simulink model "MPC_vs_LQR"  (R2014b)
settings: Solver=ode45  StartTime=0.0  StopTime=T_sim  RelTol=1e-3
values from neighbouring files (symbols this model uses):
  N = 100    [cessna.m]
  Q = eye(4)    [cessna.m]
  R = 1    [cessna.m]
  set_point = [0; 0; 0; 0]    [cessna.m]
  sys_discrete = c2d(sys, Ts)    [cessna.m]
  Ts = 0.1    [cessna.m]
  u_max_simulink = inf    [cessna.m]
  u_min_simulink = -inf    [cessna.m]
  x0 = [0; 0; 0; 10]    [cessna.m]
undefined symbols (not defined in the file or in its folder): Kdlqr, MPC_controller, S
settings Model: Creator=lele  LastModifiedBy=lele

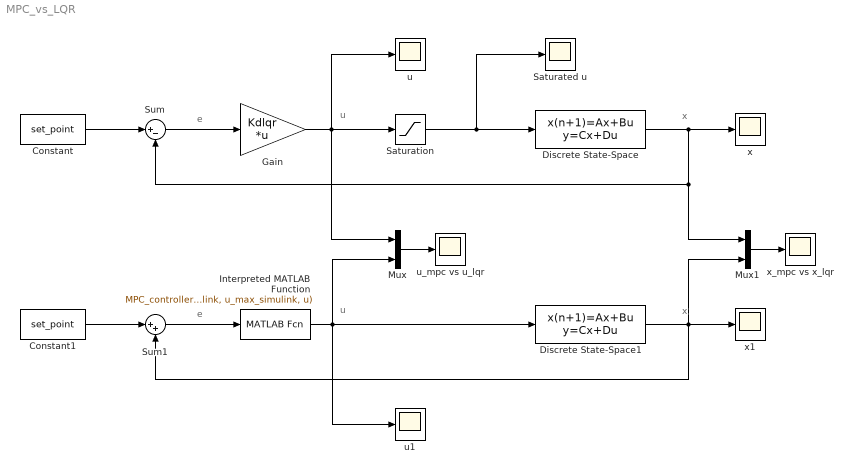
== system MPC_vs_LQR ==
  note: x
  note: u
  note: e
  note: x
  note: u
  note: e
  Constant : Constant  Value=set_point
  Constant1 : Constant  Value=set_point
  Discrete State-Space : DiscreteStateSpace  A=sys_discrete.a  B=sys_discrete.b  C=eye(4)  D=zeros(4, 1)  X0=x0  SampleTime=Ts
  Discrete State-Space1 : DiscreteStateSpace  A=sys_discrete.a  B=sys_discrete.b  C=eye(4)  D=zeros(4, 1)  X0=x0  SampleTime=Ts
  Gain : Gain  Gain=Kdlqr  Multiplication=Matrix(K*u)
  Interpreted MATLAB Function : MATLABFcn  MATLABFcn=MPC_controller(sys_discrete.a, sys_discrete.b, Q, R, S, N, u_min_simulink, u_max_simulink, u)
  Mux : Mux  Inputs=2
  Mux1 : Mux  Inputs=2
  Saturated u : Scope
      settings: SaveName=ScopeData2
  Saturation : Saturate  UpperLimit=u_max_simulink  LowerLimit=u_min_simulink
  Sum : Sum  Inputs=|+-
  Sum1 : Sum  Inputs=|++
  u : Scope
  u1 : Scope
      settings: SaveName=ScopeData4
  "u_mpc vs u_lqr " : Scope
      settings: SaveName=ScopeData3
  x : Scope
      settings: ShowLegends=on  TimeRange=10
  x1 : Scope
      settings: ShowLegends=on  SaveName=ScopeData5
  "x_mpc vs x_lqr " : Scope
      settings: ShowLegends=on  SaveName=ScopeData6
  wires:
  Constant/1 -> Sum/1
  Sum/1 -> Gain/1
  Discrete State-Space/1 -> Mux1/1, Sum/2, x/1
  Gain/1 -> Mux/1, u/1, Saturation/1
  Saturation/1 -> Discrete State-Space/1, Saturated u/1
  Constant1/1 -> Sum1/1
  Discrete State-Space1/1 -> Mux1/2, Sum1/2, x1/1
  Sum1/1 -> Interpreted MATLAB Function/1
  Interpreted MATLAB Function/1 -> Mux/2, u1/1, Discrete State-Space1/1
  Mux/1 -> "u_mpc vs u_lqr "/1
  Mux1/1 -> "x_mpc vs x_lqr "/1
